simulink model "rx_dsp_core"  (R2021a)
settings: Solver=VariableStepAuto  StartTime=0.0  StopTime=sim_time  RelTol=1e-3
values from neighbouring files (symbols this model uses):
  downsample_ratio = 8    [rx_dsp_core_init_hw.m]
  f_ddc1 = 70e6    (= 70000000)    [rx_dsp_core_init_hw.m]
  f_ddc2 = 100e6    (= 100000000)    [rx_dsp_core_init_hw.m]
  f_ddc3 = 130e6    (= 130000000)    [rx_dsp_core_init_hw.m]
  f_duc = 2.4e9    (= 2400000000)    [rx_dsp_core_init_hw.m]
  fc1 = 2.37e9    (= 2370000000)    [rx_dsp_core_init_hw.m]
  fc2 = 2.4e9    (= 2400000000)    [rx_dsp_core_init_hw.m]
  fc3 = 2.43e9    (= 2430000000)    [rx_dsp_core_init_hw.m]
  lpf1_coefficient = firpm(N, Fo, Ao, W, {dens})    [rx_dsp_core_init_hw.m]
  ts = 1/fs    (= 2.5e-10)    [rx_dsp_core_init_hw.m]
undefined symbols (not defined in the file or in its folder): designMultirateFIR
libraries: dspsrcs4 x7, dspmlti4 x3
settings Model: Creator=beheshti  LastModifiedBy=beheshti

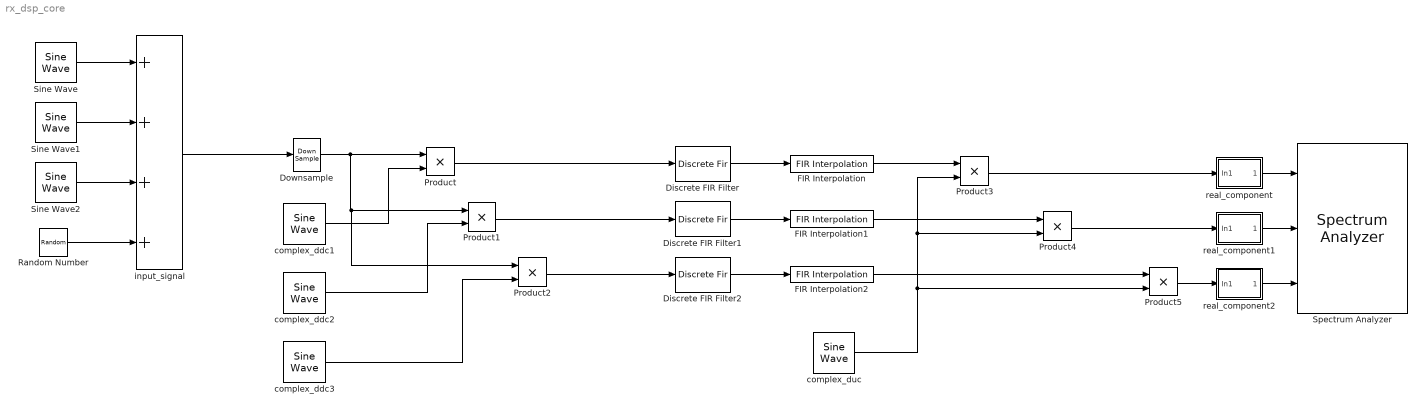
== system rx_dsp_core ==
  Discrete FIR Filter : DiscreteFir  Coefficients=lpf1_coefficient
  Discrete FIR Filter1 : DiscreteFir  Coefficients=lpf1_coefficient
  Discrete FIR Filter2 : DiscreteFir  Coefficients=lpf1_coefficient
  Downsample : DownSample  N=downsample_ratio  RateOptions=Allow multirate processing
  FIR Interpolation : dspmlti4/FIR Interpolation  FilterSource=Auto  PrivateCoeffs=0  h=designMultirateFIR(3,1)  L=downsample_ratio  FilterObject=FINTERP  framing=Allow multirate processing  outputBufInitCond=0  roundingMode=Floor  overflowMode=off  firstCoeffDataTypeStr=Inherit: Same word length as input  firstCoeffMin=[]  firstCoeffMax=[]  firstCoeffLastDataTypeStr=Inherit: Same word length as input  outputDataTypeStr=Inherit: Same as accumulator  outputMin=[]  outputMax=[]  outputLastDataTypeStr=Inherit: Same as accumulator
  FIR Interpolation1 : dspmlti4/FIR Interpolation  FilterSource=Auto  PrivateCoeffs=0  h=designMultirateFIR(3,1)  L=downsample_ratio  FilterObject=FINTERP  framing=Allow multirate processing  outputBufInitCond=0  roundingMode=Floor  overflowMode=off  firstCoeffDataTypeStr=Inherit: Same word length as input  firstCoeffMin=[]  firstCoeffMax=[]  firstCoeffLastDataTypeStr=Inherit: Same word length as input  outputDataTypeStr=Inherit: Same as accumulator  outputMin=[]  outputMax=[]  outputLastDataTypeStr=Inherit: Same as accumulator
  FIR Interpolation2 : dspmlti4/FIR Interpolation  FilterSource=Auto  PrivateCoeffs=0  h=designMultirateFIR(3,1)  L=downsample_ratio  FilterObject=FINTERP  framing=Allow multirate processing  outputBufInitCond=0  roundingMode=Floor  overflowMode=off  firstCoeffDataTypeStr=Inherit: Same word length as input  firstCoeffMin=[]  firstCoeffMax=[]  firstCoeffLastDataTypeStr=Inherit: Same word length as input  outputDataTypeStr=Inherit: Same as accumulator  outputMin=[]  outputMax=[]  outputLastDataTypeStr=Inherit: Same as accumulator
  Product{,1..5} (6 alike) : Product
  Random Number : RandomNumber  Variance=3e-5  SampleTime=ts
  Sine Wave : dspsrcs4/Sine Wave  Amplitude=1  Frequency=fc1  Phase=0  SampleMode=Discrete  OutComplex=Real  CompMethod=Trigonometric fcn  TableSize=Speed  SampleTime=ts  SamplesPerFrame=1  ResetState=Restart at time zero  OutputFrames=off  dataType=double  wordLen=16  udDataType=sfix(16)  fracBitsMode=Best precision  numFracBits=15  OutDataTypeStr=double  LastOutDataTypeStr=double
  Sine Wave1 : dspsrcs4/Sine Wave  Amplitude=2  Frequency=fc2  Phase=0  SampleMode=Discrete  OutComplex=Real  CompMethod=Trigonometric fcn  TableSize=Speed  SampleTime=ts  SamplesPerFrame=1  ResetState=Restart at time zero  OutputFrames=off  dataType=double  wordLen=16  udDataType=sfix(16)  fracBitsMode=Best precision  numFracBits=15  OutDataTypeStr=double  LastOutDataTypeStr=double
  Sine Wave2 : dspsrcs4/Sine Wave  Amplitude=3  Frequency=fc3  Phase=0  SampleMode=Discrete  OutComplex=Real  CompMethod=Trigonometric fcn  TableSize=Speed  SampleTime=ts  SamplesPerFrame=1  ResetState=Restart at time zero  OutputFrames=off  dataType=double  wordLen=16  udDataType=sfix(16)  fracBitsMode=Best precision  numFracBits=15  OutDataTypeStr=double  LastOutDataTypeStr=double
  Spectrum Analyzer : SpectrumAnalyzer  NumInputPorts=3
  complex_ddc1 : dspsrcs4/Sine Wave  Amplitude=1  Frequency=f_ddc1  Phase=0  SampleMode=Discrete  OutComplex=Complex  CompMethod=Trigonometric fcn  TableSize=Speed  SampleTime=ts*downsample_ratio  SamplesPerFrame=1  ResetState=Restart at time zero  OutputFrames=off  dataType=double  wordLen=16  udDataType=sfix(16)  fracBitsMode=Best precision  numFracBits=15  OutDataTypeStr=double  LastOutDataTypeStr=double
  complex_ddc2 : dspsrcs4/Sine Wave  Amplitude=1  Frequency=f_ddc2  Phase=0  SampleMode=Discrete  OutComplex=Complex  CompMethod=Trigonometric fcn  TableSize=Speed  SampleTime=ts*downsample_ratio  SamplesPerFrame=1  ResetState=Restart at time zero  OutputFrames=off  dataType=double  wordLen=16  udDataType=sfix(16)  fracBitsMode=Best precision  numFracBits=15  OutDataTypeStr=double  LastOutDataTypeStr=double
  complex_ddc3 : dspsrcs4/Sine Wave  Amplitude=1  Frequency=f_ddc3  Phase=0  SampleMode=Discrete  OutComplex=Complex  CompMethod=Trigonometric fcn  TableSize=Speed  SampleTime=ts*downsample_ratio  SamplesPerFrame=1  ResetState=Restart at time zero  OutputFrames=off  dataType=double  wordLen=16  udDataType=sfix(16)  fracBitsMode=Best precision  numFracBits=15  OutDataTypeStr=double  LastOutDataTypeStr=double
  complex_duc : dspsrcs4/Sine Wave  Amplitude=1  Frequency=f_duc  Phase=0  SampleMode=Discrete  OutComplex=Complex  CompMethod=Trigonometric fcn  TableSize=Speed  SampleTime=ts  SamplesPerFrame=1  ResetState=Restart at time zero  OutputFrames=off  dataType=double  wordLen=16  udDataType=sfix(16)  fracBitsMode=Best precision  numFracBits=15  OutDataTypeStr=double  LastOutDataTypeStr=double
  input_signal : Sum  Inputs=++++  AccumDataTypeStr=fixdt(1,16,0)
  real_component : Subsystem
  real_component1 : Subsystem
  real_component2 : Subsystem
  wires:
  Sine Wave/1 -> input_signal/1
  Sine Wave1/1 -> input_signal/2
  Sine Wave2/1 -> input_signal/3
  input_signal/1 -> Downsample/1
  Downsample/1 -> Product/1, Product2/1, Product1/1
  Product/1 -> Discrete FIR Filter/1
  complex_ddc1/1 -> Product/2
  complex_ddc2/1 -> Product1/2
  complex_ddc3/1 -> Product2/2
  Product1/1 -> Discrete FIR Filter1/1
  Product2/1 -> Discrete FIR Filter2/1
  Discrete FIR Filter/1 -> FIR Interpolation/1
  Discrete FIR Filter1/1 -> FIR Interpolation1/1
  Discrete FIR Filter2/1 -> FIR Interpolation2/1
  Random Number/1 -> input_signal/4
  FIR Interpolation/1 -> Product3/1
  FIR Interpolation1/1 -> Product4/1
  FIR Interpolation2/1 -> Product5/1
  Product5/1 -> real_component2/1(In1)
  Product4/1 -> real_component1/1(In1)
  Product3/1 -> real_component/1(In1)
  complex_duc/1 -> Product5/2, Product4/2, Product3/2
  real_component/1(Out1) -> Spectrum Analyzer/1
  real_component1/1(Out1) -> Spectrum Analyzer/2
  real_component2/1(Out1) -> Spectrum Analyzer/3

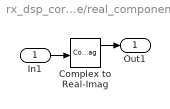
== system rx_dsp_core/real_component ==
  In1 : Inport
  Complex to Real-Imag : ComplexToRealImag
  Out1 : Outport
  wires:
  In1/1 -> Complex to Real-Imag/1
  Complex to Real-Imag/1 -> Out1/1

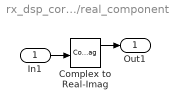
== system rx_dsp_core/real_component1 ==
  In1 : Inport
  Complex to Real-Imag : ComplexToRealImag
  Out1 : Outport
  wires:
  Complex to Real-Imag/1 -> Out1/1
  In1/1 -> Complex to Real-Imag/1

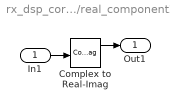
== system rx_dsp_core/real_component2 ==
  In1 : Inport
  Complex to Real-Imag : ComplexToRealImag
  Out1 : Outport
  wires:
  In1/1 -> Complex to Real-Imag/1
  Complex to Real-Imag/1 -> Out1/1
